simulink library "Condensing_Boiler_CONF"  (R2016b)
settings: Solver=ode45  StartTime=0.0  StopTime=10.0  RelTol=1e-3  EnableMultiTasking=on
undefined symbols (not defined in the file): path_carnot
libraries: carnot x1
settings Model: Creator=lena.frank  LastModifiedBy=drhf
settings DataIOCC: LimitDataPoints=on  SaveFormat=Array  SignalLoggingSaveFormat=ModelDataLogs
settings OptimizationCC: ExpressionDepthLimit=2147483647  LifeSpan=inf
settings DebuggingCC: UnderspecifiedInitializationDetection=Classic  MergeDetectMultiDrivingBlocksExec=none  SolverPrmCheckMsg=warning  FcnCallInpInsideContextMsg=warning  StateNameClashWarn=warning  SFUnexpectedBacktrackingDiag=warning  SFNoUnconditionalDefaultTransitionDiag=warning  SFExecutionAtInitializationDiag=none
settings HardwareCC: ProdBitPerPointer=32  ProdBitPerSizeT=32  ProdBitPerPtrDiffT=32  ProdLargestAtomicFloat=None  ProdIntDivRoundTo=Undefined  ProdEndianess=Unspecified  ProdWordSize=32  ProdHWDeviceType=32-bit Generic
settings ModelReferenceCC: PropagateSignalLabelsOutOfModel=off
settings GRTTargetCC: TargetLangStandard=C89/C90 (ANSI)  GeneratePreprocessorConditionals=Disable all  CombineOutputUpdateFcns=off  GRTInterface=on
settings ConfigComp: CovMetricSettings=dw  CovHtmlReporting=on  CovSaveCumulativeToWorkspaceVar=on  CovSaveSingleToWorkspaceVar=on  CovExternalEMLEnable=off

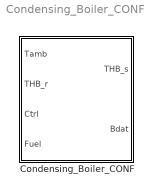
== system Condensing_Boiler_CONF ==
  Condensing_Boiler_CONF : Subsystem  mask(Configurated Condensing Boiler){Tini=20, PathName=fullfile(path_carnot('libsl'), 'Source','Boiler','Condensing_Boiler_CONF','parameter_set'), FileName='DefaultCondensingBoiler.mat', userPath=off, userParam=off, Pgas=20000, HeatLoss=2.5, Volume=0.0035, ElectricPower=[50 200], TableRelativePower=[0.1 1], whichTforEfficiency=mean of inlet and outlet temperature, TableData=[1 1;1 1], TableTemperatures=[10 90], relQdotMin=0.1, dplin=10, dpqua=100, Nodes=3}
      mask prompts: Tini "Initial temperature in °C"; PathName "Path"; FileName "Parameter set"; userPath "Edit path and name of parameter set"; userParam "User defined parameters"; Pgas "Heat input (= hi * GasMassflow) [W]"; HeatLoss "Heat losses in W/K"; Volume "Volume (of water) in m³"; ElectricPower "Electric power in W (vector, index from relative power)"; TableRelativePower "relative power in 0..1 (vector for row index)"; whichTforEfficiency "Efficiency table based on"; TableData "Efficiency data in 0..1 (matrix)"; TableTemperatures "Temperature in °C  (vector for column index)"; relQdotMin "Minimum control signal for "ON""; dplin "pressure drop linear in massflow [Pa*s/kg]"; dpqua "pressure drop quadratic in massflow [Pa*s²/kg²]"; Nodes "Number of nodes"
      mask help:
      | Multinode one-dimensional model of a boiler. Condensing effects are taken in account by an efficiency lookup table.
      | This block uses predefined parameter sets.
      mask init:
      | % callback to set parameters of model
      | [ok, param] = CarnotCallbacks_CondensingBoilerConf('SetParameters',gcbh,PathName,FileName);
      mask Help: web(fullfile(path_carnot('help'),'Condensing_Boiler_CONF.html'),'-helpbrowser')
      mask TypeOptions Tini: Condensing_Boiler/Tini
      mask Callback userPath: [ok, param] = CarnotCallbacks_CondensingBoilerConf('UserEdit',gcbh);
      mask Callback userParam: [ok, param] = CarnotCallbacks_CondensingBoilerConf('UserEdit',gcbh);
      mask TypeOptions Pgas: Condensing_Boiler/Pgas
      mask TypeOptions HeatLoss: Condensing_Boiler/UA
      mask TypeOptions Volume: Condensing_Boiler/vol
      mask TypeOptions ElectricPower: Condensing_Boiler/electricPower
      mask TypeOptions TableRelativePower: Condensing_Boiler/relativeQdot
      mask TypeOptions whichTforEfficiency: Condensing_Boiler/whichTforEfficiency
      mask TypeOptions TableData: Condensing_Boiler/efficiency
      mask TypeOptions TableTemperatures: Condensing_Boiler/temperatures
      mask TypeOptions relQdotMin: limitCtrl/relQdotMin
      mask TypeOptions dplin: Condensing_Boiler/lin
      mask TypeOptions dpqua: Condensing_Boiler/qua
      mask TypeOptions Nodes: Condensing_Boiler/nodes
      mask DialogControl Control1 Prompt: Carnot public data
      mask DialogControl Control1 Callback: [ok, file] = CarnotCallbacks_CondensingBoilerConf('GetFilename',gcbh,'public');
      mask DialogControl Control3 Prompt: Carnot internal data
      mask DialogControl Control3 Callback: [ok, file] = CarnotCallbacks_CondensingBoilerConf('GetFilename',gcbh,'internal');
      mask DialogControl Control4 Prompt: Selected path
      mask DialogControl Control4 Callback: [ok, file] = CarnotCallbacks_CondensingBoilerConf('GetFilename',gcbh,'selected');
      mask DialogControl Control5 Prompt: Save in Carnot internal data
      mask DialogControl Control5 Callback: [ok, param] = CarnotCallbacks_CondensingBoilerConf('SaveFilename',gcbh,'internal','B');
      mask DialogControl Control6 Prompt: Save in selected path
      mask DialogControl Control6 Callback: [ok, param] = CarnotCallbacks_CondensingBoilerConf('SaveFilename',gcbh,'selected','B');
      mask Display:
      | % user defined picture file
      | picfile = fullfile(path_carnot('intlibsl'), ...
      |         'Source','Boiler','Condensing_Boiler_CONF','parameter_set', ...
      |         'Condensing_Boiler_CONF.jpg');
      | 
      | pic = false;
      | if ~BlockIsInCarnotLibrary    % if not located in library any more
      |     if exist(picfile,'file') % show internal picture if defined
      |         image(imread(picfile), [0.2, 0, 0.6, 1])
      |         set_param(gcb, 'BackgroundColor', 'White')
      |         pic = true;
      |     end
      | end
      | if ~pic    % show public picture
      |     set_param(gcb, 'BackgroundColor', 'Red')
      |     plot(0,0,1,1,[10,90,90,10,10]/100,[10,10,20,20,10]/100,[80,80,20,20]/100, ...
      |         [20,90,90,20]/100,[20,70,70,20]/100,[24,24,30,30]/100,[32,30,28]/100, ...
      |         [30,40,30]/100,[43,40,38]/100,[30,40,30]/100,[53,50,47]/100, ...
      |         [30,40,30]/100,[63,60,57]/100,[30,40,30]/100, ...
      |         [35,32,30,29,31,36,39,40,37,35]/100,[75,69,65,58,50,49,53,59,68,75]/100, ...
      |         [57,54,51,51,53,58,62,62,59,57]/100,[76,71,67,58,49,48,54,60,69,76]/100)
      | end
      | 
      | % Show port labels: same as port labels in the subsystem,
      | % but display with a picture covers the text. Have to reprint it.
      | % port_label('input',1,'Tamb')
      | % port_label('input',2,'THB_r')
      | % port_label('input',3,'Ctrl')
      | % port_label('input',4,'Fuel')
      | % port_label('output',1,'THB_s')
      | % port_label('output',2,'Bdat')

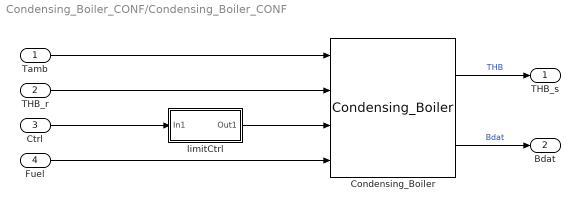
== system Condensing_Boiler_CONF/Condensing_Boiler_CONF ==
  Tamb : Inport
  THB_r : Inport  Port=2
  Ctrl : Inport  Port=3
  Fuel : Inport  Port=4
  Condensing_Boiler : carnot/Source/Boiler/Condensing_Boiler  Pgas=Pgas  UA=HeatLoss  vol=Volume  electricPower=ElectricPower  relativeQdot=TableRelativePower  whichTforEfficiency=mean of inlet and outlet temperature  temperatures=TableTemperatures  efficiency=TableData  lin=dplin  qua=dpqua  Tini=Tini  nodes=Nodes
  limitCtrl : Subsystem  mask{relQdotMin=relQdotMin}
      mask prompts: relQdotMin "Minimum control signal for "ON""
  THB_s : Outport
  Bdat : Outport  Port=2
  wires:
  Fuel/1 -> Condensing_Boiler/4
  Condensing_Boiler/2 -> Bdat/1  "Bdat"
  Condensing_Boiler/1 -> THB_s/1  "THB"
  Tamb/1 -> Condensing_Boiler/1
  THB_r/1 -> Condensing_Boiler/2
  Ctrl/1 -> limitCtrl/1(In1)
  limitCtrl/1(Out1) -> Condensing_Boiler/3

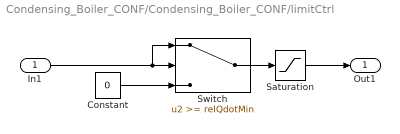
== system Condensing_Boiler_CONF/Condensing_Boiler_CONF/limitCtrl ==
  In1 : Inport
  Constant : Constant  Value=0
  Saturation : Saturate  UpperLimit=1  LowerLimit=0
  Switch : Switch  Threshold=relQdotMin
  Out1 : Outport
  wires:
  Saturation/1 -> Out1/1
  Constant/1 -> Switch/3
  Switch/1 -> Saturation/1
  In1/1 -> Switch/1, Switch/2
